simulink model "VehCtrl20260630_18B"  (R2018b)
settings: Solver=FixedStepAuto  StartTime=0.0  StopTime=inf  FixedStep=0.005  RelTol=1e-3
InitFcn:
  | mbd_mpc_consistency_checks(bdroot(gcs));
undefined symbols (not defined in the file): ANG_DEAD, BMS_NormalPwr, BrakeDeadZone, BrkPrsByBrkPct_TB_X, BrkPrsByBrkPct_TB_Y, DELAY_DISCHARGE, DELAY_RCUOFF, DRV_BACKWARD, DRV_BRAKE, DRV_FORWARD, DRV_NEUTRAL, DRV_PARK, DRV_UNPARK, DRV_ZEROTURN, EPB_LOCK, EPB_UNLOCK, ExtraLoadPwr, FanOff, fifo_0_vect, fifo_1_vect, HiFanReq, HV_finished, HV_No_Active, HV_POWER_OFF, HV_POWER_ON, HVDown, HVON, KaTLS_v_DrgUp_X_VehSpd, KeFTM_s_Way1OffDlyTime, KeFTM_TK_Way1CoolLv2OffBatTemp, KeFTM_TK_Way1CoolLv2OffMtrTemp, KeFTM_TK_Way1CoolLv2OnBatTemp, KeFTM_TK_Way1CoolLv2OnMtrTemp, KeFTM_TK_Way1CoolLv3OffBatTemp, KeFTM_TK_Way1CoolLv3OffMtrTemp, KeFTM_TK_Way1CoolLv3OnBatTemp, KeFTM_TK_Way1CoolLv3OnMtrTemp, KeFTM_TK_Way1CoolLv4OffBatTemp, KeFTM_TK_Way1CoolLv4OffMtrTemp, KeFTM_TK_Way1CoolLv4OnBatTemp, KeFTM_TK_Way1CoolLv4OnMtrTemp, Kp1, Kp2, LowFanReq, LQFP, MtrCmdGainFL, MtrCmdGainFR, MtrCmdGainRL, MtrCmdGainRR, MtrPwrFactor_RCU, MtrPwrHighToMidThd, MtrPwrLowToMidThd, MtrPwrMidToHighThd, MtrPwrMidToLowThd, MtrTrqMax, PCT_DEAD, Precharge, PTO_1000, PTO_540, pts1_fifo_0_vect ... (+32)
libraries: mbd_mpc574x_ec_toolbox x175, simulink x110, canmsglib x70
(part 7 of 15)

== system VehCtrl20260630_18B/SigOut/MCU/FL3 ==
  note: +32
  note: 0-torque
      | 1-speed
  DirCmd : Inport
  torque : Inport  Port=2
  Constant : Constant  Value=16  OutDataTypeStr=uint8
  Constant1 : Constant  Value=4  OutDataTypeStr=uint8
  Constant2 : Constant  Value=DRV_ZEROTURN  OutDataTypeStr=uint8
  Constant3 : Constant  Value=48  OutDataTypeStr=uint8
  Constant4 : Constant  Value=36  OutDataTypeStr=uint8
  Constant5 : Constant  Value=0  OutDataTypeStr=single
  Data Store Read : DataStoreRead  DataStoreName=DrvPhase
  Data Store Read1 : DataStoreRead  DataStoreName=MotorModeZeroTurn
  Data Store Read2 : DataStoreRead  DataStoreName=Gain_Trq2Spd
  GreaterThan : RelationalOperator  Operator===  OutDataTypeStr=boolean  RndMeth=Simplest
  Logical Operator : Logic  AllPortsSameDT=off  OutDataTypeStr=boolean
  NOT : Logic  Operator=NOT  IconShape=distinctive  AllPortsSameDT=off  OutDataTypeStr=boolean
  Product : Product
  Switch{,1..3} (4 alike) : Switch  Criteria=u2 > Threshold
  ModeReq : Outport
  speed : Outport  Port=2
  wires:
  DirCmd/1 -> NOT/1
  Constant/1 -> Switch/1
  Constant1/1 -> Switch/3
  Data Store Read/1 -> GreaterThan/1
  Constant2/1 -> GreaterThan/2
  GreaterThan/1 -> Logical Operator/1
  Data Store Read1/1 -> Logical Operator/2
  Logical Operator/1 -> Switch3/2, Switch1/2
  Switch/1 -> Switch1/3
  Switch1/1 -> ModeReq/1
  NOT/1 -> Switch2/2, Switch/2
  Constant4/1 -> Switch2/3
  Constant3/1 -> Switch2/1
  Switch2/1 -> Switch1/1
  torque/1 -> Product/2
  Switch3/1 -> speed/1
  Product/1 -> Switch3/1
  Data Store Read2/1 -> Product/1
  Constant5/1 -> Switch3/3

== system VehCtrl20260630_18B/SigOut/MCU/FR ==
  DirCmd : Inport
  Constant : Constant  Value=16  OutDataTypeStr=uint8
  Constant1 : Constant  Value=4  OutDataTypeStr=uint8
  NOT : Logic  Operator=NOT  IconShape=distinctive  AllPortsSameDT=off  OutDataTypeStr=boolean
  Switch : Switch  Criteria=u2 > Threshold
  ModeReq : Outport
  wires:
  Switch/1 -> ModeReq/1
  NOT/1 -> Switch/2
  Constant1/1 -> Switch/3
  Constant/1 -> Switch/1
  DirCmd/1 -> NOT/1

== system VehCtrl20260630_18B/SigOut/MCU/RL ==
  DirCmd : Inport
  Constant : Constant  Value=16  OutDataTypeStr=uint8
  Constant1 : Constant  Value=4  OutDataTypeStr=uint8
  Switch : Switch  Criteria=u2 > Threshold
  ModeReq : Outport
  wires:
  Constant/1 -> Switch/1
  Constant1/1 -> Switch/3
  DirCmd/1 -> Switch/2
  Switch/1 -> ModeReq/1

== system VehCtrl20260630_18B/SigOut/MCU/RR ==
  DirCmd : Inport
  Constant : Constant  Value=16  OutDataTypeStr=uint8
  Constant1 : Constant  Value=4  OutDataTypeStr=uint8
  NOT : Logic  Operator=NOT  IconShape=distinctive  AllPortsSameDT=off  OutDataTypeStr=boolean
  Switch : Switch  Criteria=u2 > Threshold
  ModeReq : Outport
  wires:
  Switch/1 -> ModeReq/1
  NOT/1 -> Switch/2
  Constant1/1 -> Switch/3
  Constant/1 -> Switch/1
  DirCmd/1 -> NOT/1

== system VehCtrl20260630_18B/SigOut/MCU/Subsystem ==
  <TrqCmd> : Inport
  Abs : Abs
  Add : Sum
  Constant : Constant  Value=MtrCmdGainFL
  Product : Product
  Saturation : Saturate  UpperLimit=100  LowerLimit=2
  Out1 : Outport
  wires:
  Abs/1 -> Add/1
  <TrqCmd>/1 -> Saturation/1, Abs/1
  Add/1 -> Out1/1
  Saturation/1 -> Product/1
  Product/1 -> Add/2
  Constant/1 -> Product/2  "MtrCmdGainFL"

== system VehCtrl20260630_18B/SigOut/MCU/Subsystem1 ==
  <TrqCmd> : Inport
  Abs : Abs
  Add : Sum
  Constant : Constant  Value=MtrCmdGainFR
  Product : Product
  Saturation : Saturate  UpperLimit=100  LowerLimit=2
  Out1 : Outport
  wires:
  Abs/1 -> Add/1
  <TrqCmd>/1 -> Saturation/1, Abs/1
  Add/1 -> Out1/1
  Saturation/1 -> Product/1
  Product/1 -> Add/2
  Constant/1 -> Product/2  "MtrCmdGainFR"

== system VehCtrl20260630_18B/SigOut/MCU/Subsystem2 ==
  <TrqCmd> : Inport
  Abs : Abs
  Add : Sum
  Constant : Constant  Value=MtrCmdGainRL
  Product : Product
  Saturation : Saturate  UpperLimit=100  LowerLimit=2
  Out1 : Outport
  wires:
  Abs/1 -> Add/1
  <TrqCmd>/1 -> Saturation/1, Abs/1
  Add/1 -> Out1/1
  Saturation/1 -> Product/1
  Product/1 -> Add/2
  Constant/1 -> Product/2  "MtrCmdGainRL"

== system VehCtrl20260630_18B/SigOut/MCU/Subsystem3 ==
  <TrqCmd> : Inport
  Abs : Abs
  Add : Sum
  Constant : Constant  Value=MtrCmdGainRR
  Product : Product
  Saturation : Saturate  UpperLimit=100  LowerLimit=2
  Out1 : Outport
  wires:
  Abs/1 -> Add/1
  <TrqCmd>/1 -> Saturation/1, Abs/1
  Add/1 -> Out1/1
  Saturation/1 -> Product/1
  Product/1 -> Add/2
  Constant/1 -> Product/2  "MtrCmdGainRR"

== system VehCtrl20260630_18B/SigOut/METER/Subsystem ==
  <ModeDir> : Inport
  Constant : Constant  Value=3
  Constant18 : Constant  Value=2
  Data Type Conversion : DataTypeConversion
  Data Type Conversion1 : DataTypeConversion
  Switch : Switch  Criteria=u2 > Threshold
  Out1 : Outport
  wires:
  Constant/1 -> Data Type Conversion/1
  Switch/1 -> Out1/1
  Constant18/1 -> Data Type Conversion1/1
  <ModeDir>/1 -> Switch/2
  Data Type Conversion/1 -> Switch/1
  Data Type Conversion1/1 -> Switch/3

== system VehCtrl20260630_18B/SigOut/METER/Subsystem1 ==
  <RCU_ActWorkSts> : Inport
  Constant : Constant
  Constant1 : Constant  Value=0
  Switch : Switch  Criteria=u2 > Threshold  Threshold=2
  Out1 : Outport
  wires:
  <RCU_ActWorkSts>/1 -> Switch/2
  Constant1/1 -> Switch/3
  Constant/1 -> Switch/1
  Switch/1 -> Out1/1

== system VehCtrl20260630_18B/SigOut/METER/Subsystem2 ==
  <DCDC_Optvol> : Inport
  Constant2 : Constant  Value=12.5
  Data Type Conversion : DataTypeConversion
  Equal : RelationalOperator  Operator=<=  OutDataTypeStr=boolean  RndMeth=Simplest
  Out1 : Outport
  wires:
  Constant2/1 -> Data Type Conversion/1
  Equal/1 -> Out1/1
  <DCDC_Optvol>/1 -> Equal/1
  Data Type Conversion/1 -> Equal/2

== system VehCtrl20260630_18B/SigOut/METER/Subsystem3 ==
  Constant : Constant  Value=2
  Constant1 : Constant
  Data Store Read1 : DataStoreRead  DataStoreName=CtrMode
  Data Store Read2 : DataStoreRead  DataStoreName=Fault
  Data Type Conversion : DataTypeConversion
  Data Type Conversion1 : DataTypeConversion
  Data Type Conversion2 : DataTypeConversion
  Equal : RelationalOperator  Operator===  OutDataTypeStr=boolean  RndMeth=Simplest
  Switch : Switch  Criteria=u2 > Threshold
  Out1 : Outport
  wires:
  Switch/1 -> Data Type Conversion1/1
  Data Store Read2/1 -> Switch/2
  Data Store Read1/1 -> Data Type Conversion/1
  Constant/1 -> Switch/1
  Data Type Conversion/1 -> Switch/3
  Data Type Conversion1/1 -> Equal/1
  Constant1/1 -> Data Type Conversion2/1
  Data Type Conversion2/1 -> Equal/2
  Equal/1 -> Out1/1

== system VehCtrl20260630_18B/SigOut/METER/Subsystem4 ==
  Constant : Constant  Value=2
  Constant1 : Constant  Value=0
  Data Store Read1 : DataStoreRead  DataStoreName=CtrMode
  Data Store Read2 : DataStoreRead  DataStoreName=Fault
  Data Type Conversion : DataTypeConversion
  Data Type Conversion1 : DataTypeConversion
  Data Type Conversion2 : DataTypeConversion
  Equal : RelationalOperator  Operator===  OutDataTypeStr=boolean  RndMeth=Simplest
  Switch : Switch  Criteria=u2 > Threshold
  Out1 : Outport
  wires:
  Switch/1 -> Data Type Conversion1/1
  Data Store Read2/1 -> Switch/2
  Data Store Read1/1 -> Data Type Conversion/1
  Constant/1 -> Switch/1
  Data Type Conversion/1 -> Switch/3
  Data Type Conversion1/1 -> Equal/1
  Constant1/1 -> Data Type Conversion2/1
  Data Type Conversion2/1 -> Equal/2
  Equal/1 -> Out1/1

== system VehCtrl20260630_18B/VehCtrl/EnergyManage1/Subsystem ==
  VehTrqTgt : Inport
  VehSpd : Inport  Port=2
  MCU_PTO : Inport  Port=3
  Add : Sum
  Bus Selector3 : BusSelector  OutputSignals=MCU2VCU_1.MCU_TrqEst,MCU2VCU_1.MCU_SpdEst
  Constant2 : Constant  Value=WhlRadius
  Constant3 : Constant  Value=9.55  OutDataTypeStr=single
  Divide : Product  Inputs=*/
  Divide1 : Product  Inputs=*/
  Product : Product
  Product1 : Product
  PwrCmd : Outport
  wires:
  Constant3/1 -> Divide1/2
  Divide/1 -> Product/2
  Product/1 -> Add/1
  Constant2/1 -> Divide/2
  Bus Selector3/2 -> Divide1/1  "<MCU_SpdEst>"
  Divide1/1 -> Product1/2
  Product1/1 -> Add/2
  Bus Selector3/1 -> Product1/1  "<MCU_TrqEst>"
  VehTrqTgt/1 -> Product/1
  VehSpd/1 -> Divide/1
  Add/1 -> PwrCmd/1
  MCU_PTO/1 -> Bus Selector3/1

== system VehCtrl20260630_18B/VehCtrl/FaultProc/Subsystem5 ==
  note: 1-正常
      | 0-超时
  note: 1-丢包
      | 0-正常
  AutoDrive : Inport
  Bus Selector7 : BusSelector  OutputSignals=signal1.AUTO_LiveCnt1,signal1.AUTO_CheckSum1,signal1.PacketLossFlg,signal2.AUTO_LiveCnt2,signal2.AUTO_CheckSum2,signal2.PacketLossFlg,signal3.AUTO_LiveCnt1,signal3.AUTO_CheckSum1,signal3.PacketLossFlg
  Logical Operator : Logic  Operator=NOT  AllPortsSameDT=off  OutDataTypeStr=boolean
  Logical Operator1 : Logic  Operator=OR  Inputs=3  AllPortsSameDT=off  OutDataTypeStr=boolean
  Logical Operator2 : Logic  Inputs=3  AllPortsSameDT=off  OutDataTypeStr=boolean
  PacketLoss_RMT : Stateflow chart  TreatAsAtomicUnit=on
  PacketLoss_RMT1 : Stateflow chart  TreatAsAtomicUnit=on
  PacketLoss_RMT2 : Stateflow chart  TreatAsAtomicUnit=on
  TimeOutLevel_RMT : Stateflow chart  TreatAsAtomicUnit=on
  TimeOutLevel_RMT1 : Stateflow chart  TreatAsAtomicUnit=on
  TimeOutLevel_RMT2 : Stateflow chart  TreatAsAtomicUnit=on
  TimeOut : Outport
  PacketLoss : Outport  Port=2
  wires:
  TimeOutLevel_RMT/1(TimeOutLevel) -> Logical Operator2/1  "TimeOutLevel1"
  Logical Operator2/1 -> Logical Operator/1
  [Auto_LiveCounter] -> TimeOutLevel_RMT/1(LiveCounter)
  Logical Operator1/1 -> PacketLoss/1
  [Auto_PacketLossFlg] -> PacketLoss_RMT/2(PacketLoss)
  [Auto_CheckSumFlg] -> PacketLoss_RMT/1(CheckSum)
  PacketLoss_RMT/1(PacketLossFlg) -> Logical Operator1/1
  AutoDrive/1 -> Bus Selector7/1
  Logical Operator/1 -> TimeOut/1
  [Auto_LiveCounter2] -> TimeOutLevel_RMT1/1(LiveCounter)
  TimeOutLevel_RMT1/1(TimeOutLevel) -> Logical Operator2/2  "TimeOutLevel1"
  [Auto_CheckSumFlg2] -> PacketLoss_RMT1/1(CheckSum)
  [Auto_PacketLossFlg2] -> PacketLoss_RMT1/2(PacketLoss)
  PacketLoss_RMT1/1(PacketLossFlg) -> Logical Operator1/2
  Bus Selector7/6 -> [Auto_PacketLossFlg2]  "<PacketLossFlg>"
  Bus Selector7/5 -> [Auto_CheckSumFlg2]  "<AUTO_CheckSum2>"
  Bus Selector7/4 -> [Auto_LiveCounter2]  "<AUTO_LiveCnt2>"
  Bus Selector7/3 -> [Auto_PacketLossFlg]  "<PacketLossFlg>"
  Bus Selector7/2 -> [Auto_CheckSumFlg]  "<AUTO_CheckSum1>"
  Bus Selector7/1 -> [Auto_LiveCounter]  "<AUTO_LiveCnt1>"
  Bus Selector7/7 -> [Auto_LiveCounter3]  "<AUTO_LiveCnt1>"
  Bus Selector7/8 -> [Auto_CheckSumFlg3]  "<AUTO_CheckSum1>"
  Bus Selector7/9 -> [Auto_PacketLossFlg3]  "<PacketLossFlg>"
  [Auto_LiveCounter3] -> TimeOutLevel_RMT2/1(LiveCounter)
  TimeOutLevel_RMT2/1(TimeOutLevel) -> Logical Operator2/3  "TimeOutLevel1"
  [Auto_PacketLossFlg3] -> PacketLoss_RMT2/2(PacketLoss)
  [Auto_CheckSumFlg3] -> PacketLoss_RMT2/1(CheckSum)
  PacketLoss_RMT2/1(PacketLossFlg) -> Logical Operator1/3

== system VehCtrl20260630_18B/VehCtrl/MontionControl/DriveControl ==
  EN_COM : Inport
  Ready : Inport  Port=2
  Fault : Inport  Port=3
  CMD : Inport  Port=4
  BMS : Inport  Port=5
  VehSpd : Inport  Port=6
  StrReady : Inport  Port=7
  AUTO : Inport  Port=8
  AUTOMode : Inport  Port=9
  RMT : Inport  Port=10
  DCDC : Inport  Port=11
  Brake : Subsystem
  Bus Creator{1..4} (4 alike) : BusCreator  Inputs=4
  Bus Selector : BusSelector  OutputSignals=RMT.RMT1.RMT_CmdAccPct,BrkPct,ModeDir,ModeStr,StrAng,RMT.RMT4.ModeSafety
  Constant : Constant  Value=0  OutDataTypeStr=uint8
  Constant1 : Constant
  Constant2 : Constant  Value=0  OutDataTypeStr=uint8
  Constant3 : Constant  OutDataTypeStr=boolean
  DriveModeTrans : Stateflow chart  TreatAsAtomicUnit=on
  Equal : RelationalOperator  Operator===  OutDataTypeStr=boolean  RndMeth=Simplest
  Logical Operator : Logic  AllPortsSameDT=off  OutDataTypeStr=boolean
  Motor : Subsystem
  MCUFL_OUT : Outport
  MCUFR_OUT : Outport  Port=2
  MCURL_OUT : Outport  Port=3
  MCURR_OUT : Outport  Port=4
  BrkPrsTgt : Outport  Port=5
  EpbSt : Outport  Port=6
  VehTrqTgt : Outport  Port=7
  wires:
  CMD/1 -> Bus Selector/1
  Bus Selector/3 -> DriveModeTrans/5(ModeDirection)  "<ModeDir>"
  Bus Selector/2 -> DriveModeTrans/2(CmdBrk)  "<BrkPct>"
  Brake/1(BrkPrsTgt) -> BrkPrsTgt/1
  DriveModeTrans/1(VehBrk) -> Brake/1(VehBrkTgt)
  DriveModeTrans/2(EpbSt) -> EpbSt/1
  VehSpd/1 -> DriveModeTrans/9(VehSpd), Motor/5(VehSpd)
  DriveModeTrans/3(VehDrv) -> Motor/1(VehDrvPct)
  Bus Selector/1 -> DriveModeTrans/1(CmdDrv)  "<RMT_CmdAccPct>"
  Bus Selector/4 -> Logical Operator/1  "<ModeStr>"
  StrReady/1 -> DriveModeTrans/8(StrReady)
  DriveModeTrans/4(SpdTgt) -> Motor/2(CmdSpd)
  DriveModeTrans/5(ModeSpd) -> Motor/3(ModeSpeed)
  DriveModeTrans/6(DrvPhase) -> Motor/4(DrvPhase)
  Bus Selector/5 -> Motor/6(CmdStrAng)  "<StrAng>"
  Motor/2(MtrDirCmdFL) -> Bus Creator1/2  "DirCmd"
  Motor/1(Enable) -> Bus Creator1/1, Bus Creator2/1, Bus Creator4/1, Bus Creator3/1  "Enable"
  Bus Creator4/1 -> MCURR_OUT/1
  Bus Creator2/1 -> MCUFR_OUT/1
  Motor/13(MtrSpdCmdRR) -> Bus Creator4/4  "SpdCmd"
  Motor/12(MtrTrqCmdRR) -> Bus Creator4/3  "TrqCmd"
  Motor/11(MtrDirCmdRR) -> Bus Creator4/2  "DirCmd"
  Bus Creator1/1 -> MCUFL_OUT/1
  Motor/7(MtrSpdCmdFR) -> Bus Creator2/4  "SpdCmd"
  Motor/6(MtrTrqCmdFR) -> Bus Creator2/3  "TrqCmd"
  Bus Creator3/1 -> MCURL_OUT/1
  Motor/10(MtrSpdCmdRL) -> Bus Creator3/4  "SpdCmd"
  Motor/4(MtrSpdCmdFL) -> Bus Creator1/4  "SpdCmd"
  Motor/9(MtrTrqCmdRL) -> Bus Creator3/3  "TrqCmd"
  Motor/3(MtrTrqCmdFL) -> Bus Creator1/3  "TrqCmd"
  Motor/8(MtrDirCmdRL) -> Bus Creator3/2  "DirCmd"
  Motor/5(MtrDirCmdFR) -> Bus Creator2/2  "DirCmd"
  Ready/1 -> Motor/9(Ready)
  Motor/14(VehTrqTgt) -> VehTrqTgt/1
  Constant/1 -> DriveModeTrans/3(ModeDrive)
  Constant1/1 -> DriveModeTrans/4(CmdPark)
  Constant2/1 -> DriveModeTrans/7(CmdSpd)
  Bus Selector/6 -> Equal/1, Motor/7(ModeSafety)  "<ModeSafety>"
  AUTO/1 -> Motor/10(AUTO)
  AUTOMode/1 -> Motor/11(AUTOMode)
  BMS/1 -> Motor/12(BMS)
  RMT/1 -> Motor/13(RMT)
  DCDC/1 -> Motor/14(DCDC)
  Fault/1 -> Brake/2(In2), Motor/8(Fault)
  Logical Operator/1 -> DriveModeTrans/6(ModeSteer)
  Equal/1 -> Logical Operator/2
  Constant3/1 -> Equal/2
  EN_COM/1 -> Motor/15(EN_COM)

== system VehCtrl20260630_18B/VehCtrl/MontionControl/PtoControl ==
  CMD : Inport
  Fault : Inport  Port=2
  Ready : Inport  Port=3
  AUTOMode : Inport  Port=4
  AUTO : Inport  Port=5
  Bus Creator : BusCreator  Inputs=4
  Bus Selector : BusSelector  OutputSignals=ShutDown,NonDrive,NonPto
  Bus Selector1 : BusSelector  OutputSignals=RMT.RMT4.RMT_PtoMode
  Bus Selector2 : BusSelector  OutputSignals=signal2.AUTO_PtoSpd
  Constant5 : Constant  Value=0  OutDataTypeStr=single
  Constant6 : Constant  OutDataTypeStr=uint8
  Constant7 : Constant  Value=0  OutDataTypeStr=uint8
  Logical Operator : Logic  Operator=OR  Inputs=3  AllPortsSameDT=off  OutDataTypeStr=boolean
  Logical Operator1 : Logic  AllPortsSameDT=off  OutDataTypeStr=boolean
  NOT : Logic  Operator=NOT  IconShape=distinctive  AllPortsSameDT=off  OutDataTypeStr=boolean
  Subsystem : Subsystem
  Subsystem1 : Subsystem
  Switch2 : Switch  Criteria=u2 > Threshold
  MCU_PTO_OUT : Outport
  wires:
  CMD/1 -> Bus Selector1/1
  Constant5/1 -> Bus Creator/3  "MtrTrqCmd"
  Subsystem/1(ModeReq) -> Bus Creator/1  "ModeReq"
  Constant6/1 -> Subsystem/1(ModeSpeed)
  Constant7/1 -> Subsystem/2(DirCmd)
  Fault/1 -> Bus Selector/1
  Bus Selector/1 -> Logical Operator/1  "<ShutDown>"
  Bus Selector/2 -> Logical Operator/2  "<NonDrive>"
  Bus Selector/3 -> Logical Operator/3  "<NonPto>"
  Logical Operator/1 -> NOT/1
  Ready/1 -> Logical Operator1/2
  NOT/1 -> Logical Operator1/1
  Logical Operator1/1 -> Bus Creator/4  "Enable"
  Bus Creator/1 -> MCU_PTO_OUT/1
  AUTOMode/1 -> Switch2/2
  Bus Selector1/1 -> Subsystem1/1(<RMT_PtoMode>)  "<RMT_PtoMode>"
  AUTO/1 -> Bus Selector2/1
  Bus Selector2/1 -> Switch2/1  "<AUTO_PtoSpd>"
  Switch2/1 -> Bus Creator/2  "MtrSpdCmd"
  Subsystem1/1(MtrSpdCmd) -> Switch2/3

== system VehCtrl20260630_18B/VehCtrl/MontionControl/SteerControl ==
  note: 这个是模式，不是方向
  VehSpd : Inport
  CMD : Inport  Port=2
  BDX : Inport  Port=3
  Bus Selector : BusSelector  OutputSignals=ModeStr,StrAng
  Bus Selector1 : BusSelector  OutputSignals=AVCU.BDX_SteeringAngle
  Chart : Stateflow chart  TreatAsAtomicUnit=on
  Constant2 : Constant  Value=10  OutDataTypeStr=uint8
  GreaterThan : RelationalOperator  Operator=<  OutDataTypeStr=boolean  RndMeth=Simplest
  StrReady : Outport
  AngCmd : Outport  Port=2
  wires:
  CMD/1 -> Bus Selector/1
  Bus Selector/1 -> Chart/2(Mode)  "<ModeStr>"
  Bus Selector/2 -> Chart/3(AngCmd)  "<StrAng>"
  BDX/1 -> Bus Selector1/1
  Bus Selector1/1 -> Chart/4(Ang)  "<BDX_SteeringAngle>"
  Chart/2(StrPhase) -> GreaterThan/1
  GreaterThan/1 -> StrReady/1
  Constant2/1 -> GreaterThan/2
  VehSpd/1 -> Chart/1(VehSpd)
  Chart/1(AngCmdOut) -> AngCmd/1

== system VehCtrl20260630_18B/VehCtrl/MontionControl/ValveControl ==
  note: 仅在安全模式下才能控制
  BrkPrsTgt : Inport
  EpbSt : Inport  Port=2
  BDX : Inport  Port=3
  CMD : Inport  Port=4
  Ready : Inport  Port=5
  "AngCmd " : Inport  Port=6
  fault : Inport  Port=7
  VehSpd : Inport  Port=8
  BrakeSys : Subsystem
  Bus Creator : BusCreator  Inputs=9
  Bus Selector : BusSelector  OutputSignals=ModeSusp,RMT.RMT4.ModeSafety,RMT.RMT2.RMT_ModeWidth
  Bus Selector1 : BusSelector  OutputSignals=AVCU.BDX_BrakePressure
  Bus Selector2 : BusSelector  OutputSignals=NonDrive
  EpbSys : Subsystem
  PumpSys : Subsystem
  SteerSys : Subsystem
  SuspesionSys : Subsystem
  WidthSys : Subsystem
  BDX_OUT : Outport
  wires:
  CMD/1 -> Bus Selector/1
  BDX/1 -> Bus Selector1/1
  BrkPrsTgt/1 -> BrakeSys/1(BrkPrsTgt)
  Bus Selector1/1 -> BrakeSys/2(BrkPrs)  "<BDX_BrakePressure>"
  Bus Selector/1 -> SuspesionSys/1(SuspSt)  "<ModeSusp>"
  Bus Selector/3 -> WidthSys/2(<RMT_ModeWidth>)  "<RMT_ModeWidth>"
  BrakeSys/1(BrkValve) -> Bus Creator/2  "BrkValve"
  SuspesionSys/1(SuspUpValve) -> Bus Creator/6  "SuspUpValve"
  PumpSys/1(Pump) -> Bus Creator/1  "Pump"
  EpbSys/1(EpbValve) -> Bus Creator/5  "EpbValve"
  SteerSys/1(SteerValveL) -> Bus Creator/3  "SteerValveL"
  WidthSys/1(WidthLengthenValve) -> Bus Creator/8  "WidthLengthenValve"
  WidthSys/2(WidthShortenValve) -> Bus Creator/9  "WidthShortenValve"
  Bus Creator/1 -> BDX_OUT/1
  SteerSys/2(SteerValveR) -> Bus Creator/4  "SteerValveR"
  EpbSt/1 -> EpbSys/1(EpbSt)
  SuspesionSys/2(SuspDownValve) -> Bus Creator/7  "SuspDownValve"
  Ready/1 -> PumpSys/1(Ready)
  Bus Selector/2 -> WidthSys/1(ModeSafety), SuspesionSys/2(ModeSafety)  "<ModeSafety>"
  fault/1 -> Bus Selector2/1
  Bus Selector2/1 -> SteerSys/2(In2)  "<NonDrive>"
  VehSpd/1 -> SteerSys/3(VehSpd)
  "AngCmd "/1 -> SteerSys/1(AngCmd)

== system VehCtrl20260630_18B/VehCtrl/TempertureControl/Lv_to_Dut1 ==
  note: 就是整型，不要替换为single
  MCUReqMtrPumpLv : Inport
  2-D Lookup Table1 : Lookup_n-D  NumberOfTableDimensions=1  BreakpointsForDimension1=uint8([ 0 1 2 3 4 ])  BreakpointsForDimension2=KaTLS_v_DrgUp_X_VehSpd  Table=uint16([ 5 30 40 55 70])  TableDataTypeStr=uint16  ExtrapMethod=Clip  UseLastTableValue=on  OutDataTypeStr=Inherit: Inherit from 'Table data'  RndMeth=Simplest
  Gain : Gain  Gain=1/100  OutDataTypeStr=single
  MCUReqMtrPumpDut : Outport
  wires:
  MCUReqMtrPumpLv/1 -> 2-D Lookup Table1/1
  2-D Lookup Table1/1 -> Gain/1
  Gain/1 -> MCUReqMtrPumpDut/1

== system VehCtrl20260630_18B/VehCtrl/TempertureControl/Lv_to_Dut2 ==
  note: 就是整型，不要替换为single
  MCUReqMtrPumpLv : Inport
  2-D Lookup Table1 : Lookup_n-D  NumberOfTableDimensions=1  BreakpointsForDimension1=uint8([ 0 1 2 3 4 ])  BreakpointsForDimension2=KaTLS_v_DrgUp_X_VehSpd  Table=uint16([ 5 30 40 55 70])  TableDataTypeStr=uint16  ExtrapMethod=Clip  UseLastTableValue=on  OutDataTypeStr=Inherit: Inherit from 'Table data'  RndMeth=Simplest
  Gain : Gain  Gain=1/100  OutDataTypeStr=single
  MCUReqMtrPumpDut : Outport
  wires:
  MCUReqMtrPumpLv/1 -> 2-D Lookup Table1/1
  2-D Lookup Table1/1 -> Gain/1
  Gain/1 -> MCUReqMtrPumpDut/1

== system VehCtrl20260630_18B/VehCtrl/TempertureControl/Lv_to_Dut3 ==
  note: 就是整型，不要替换为single
  MCUReqBatPumpLv : Inport
  2-D Lookup Table1 : Lookup_n-D  NumberOfTableDimensions=1  BreakpointsForDimension1=uint8([ 0 1 2 3 4 ])  BreakpointsForDimension2=KaTLS_v_DrgUp_X_VehSpd  Table=uint16([ 5 30 40 55 70])  TableDataTypeStr=uint16  ExtrapMethod=Clip  UseLastTableValue=on  OutDataTypeStr=Inherit: Inherit from 'Table data'  RndMeth=Simplest
  Gain : Gain  Gain=1/100  OutDataTypeStr=single
  MCUReqBatPumpDut : Outport
  wires:
  MCUReqBatPumpLv/1 -> 2-D Lookup Table1/1
  2-D Lookup Table1/1 -> Gain/1
  Gain/1 -> MCUReqBatPumpDut/1

== system VehCtrl20260630_18B/VehCtrl/TempertureControl/ThermFR_RRvRead1 ==
  RdySt : Inport
  MtrTemp : Inport  Port=2
  Cnt_To_s : Subsystem
  Constant10 : Constant  Value=KeFTM_TK_Way1CoolLv3OnMtrTemp
  Constant11 : Constant  Value=KeFTM_TK_Way1CoolLv2OffMtrTemp
  Constant12 : Constant  Value=KeFTM_TK_Way1CoolLv2OnMtrTemp
  Constant13 : Constant  Value=KeFTM_TK_Way1CoolLv4OnMtrTemp
  Constant7 : Constant  Value=KeFTM_s_Way1OffDlyTime
  Constant8 : Constant  Value=KeFTM_TK_Way1CoolLv4OffMtrTemp
  Constant9 : Constant  Value=KeFTM_TK_Way1CoolLv3OffMtrTemp
  Way1_Cool_Level : Stateflow chart  TreatAsAtomicUnit=on
  MtrPumpLvReq : Outport
  Fan_Low : Outport  Port=2
  wires:
  Way1_Cool_Level/2(MtrPumpLv) -> MtrPumpLvReq/1  "MtrPumpLvReq2"
  Way1_Cool_Level/1(Fan_Low) -> Fan_Low/1  "FanLvReq2"
  RdySt/1 -> Way1_Cool_Level/1(RdySt)
  Constant13/1 -> Way1_Cool_Level/8(Ke_Lv4OnTemp)
  Constant12/1 -> Way1_Cool_Level/4(Ke_Lv2OnTemp)
  Constant10/1 -> Way1_Cool_Level/6(Ke_Lv3OnTemp)
  Constant9/1 -> Way1_Cool_Level/5(Ke_Lv3OffTemp)
  Constant11/1 -> Way1_Cool_Level/3(Ke_Lv2OffTemp)
  Constant7/1 -> Cnt_To_s/1(In1)
  Constant8/1 -> Way1_Cool_Level/7(Ke_Lv4OffTemp)
  Cnt_To_s/1(Out1) -> Way1_Cool_Level/9(Ke_OffDlyCnt)
  MtrTemp/1 -> Way1_Cool_Level/2(Temp)

== system VehCtrl20260630_18B/VehCtrl/TempertureControl/ThermFR_RRvRead2 ==
  RdySt : Inport
  MtrTemp : Inport  Port=2
  Cnt_To_s : Subsystem
  Constant10 : Constant  Value=KeFTM_TK_Way1CoolLv3OnMtrTemp
  Constant11 : Constant  Value=KeFTM_TK_Way1CoolLv2OffMtrTemp
  Constant12 : Constant  Value=KeFTM_TK_Way1CoolLv2OnMtrTemp
  Constant13 : Constant  Value=KeFTM_TK_Way1CoolLv4OnMtrTemp
  Constant7 : Constant  Value=KeFTM_s_Way1OffDlyTime
  Constant8 : Constant  Value=KeFTM_TK_Way1CoolLv4OffMtrTemp
  Constant9 : Constant  Value=KeFTM_TK_Way1CoolLv3OffMtrTemp
  Way1_Cool_Level : Stateflow chart  TreatAsAtomicUnit=on
  MtrPumpLvReq : Outport
  Fan_Low : Outport  Port=2
  wires:
  MtrTemp/1 -> Way1_Cool_Level/2(Temp)
  Cnt_To_s/1(Out1) -> Way1_Cool_Level/9(Ke_OffDlyCnt)
  Constant8/1 -> Way1_Cool_Level/7(Ke_Lv4OffTemp)
  Constant7/1 -> Cnt_To_s/1(In1)
  Constant11/1 -> Way1_Cool_Level/3(Ke_Lv2OffTemp)
  Constant9/1 -> Way1_Cool_Level/5(Ke_Lv3OffTemp)
  Constant10/1 -> Way1_Cool_Level/6(Ke_Lv3OnTemp)
  Constant12/1 -> Way1_Cool_Level/4(Ke_Lv2OnTemp)
  Constant13/1 -> Way1_Cool_Level/8(Ke_Lv4OnTemp)
  RdySt/1 -> Way1_Cool_Level/1(RdySt)
  Way1_Cool_Level/1(Fan_Low) -> Fan_Low/1  "FanLvReq2"
  Way1_Cool_Level/2(MtrPumpLv) -> MtrPumpLvReq/1  "MtrPumpLvReq2"

== system VehCtrl20260630_18B/VehCtrl/TempertureControl/ThermLvRead3 ==
  RdySt : Inport
  Temp : Inport  Port=2
  Cnt_To_s : Subsystem
  Constant10 : Constant  Value=KeFTM_TK_Way1CoolLv3OnBatTemp
  Constant11 : Constant  Value=KeFTM_TK_Way1CoolLv2OffBatTemp
  Constant12 : Constant  Value=KeFTM_TK_Way1CoolLv2OnBatTemp
  Constant13 : Constant  Value=KeFTM_TK_Way1CoolLv4OnBatTemp
  Constant7 : Constant  Value=KeFTM_s_Way1OffDlyTime
  Constant8 : Constant  Value=KeFTM_TK_Way1CoolLv4OffBatTemp
  Constant9 : Constant  Value=KeFTM_TK_Way1CoolLv3OffBatTemp
  Way1_Cool_Level : Stateflow chart  TreatAsAtomicUnit=on
  Fan_Low : Outport
  Fan_High : Outport  Port=2
  v1 : Outport  Port=3
  v2 : Outport  Port=4
  v3 : Outport  Port=5
  v4 : Outport  Port=6
  PumpLvReq : Outport  Port=7
  wires:
  Way1_Cool_Level/2(Fan_High) -> Fan_High/1
  Temp/1 -> Way1_Cool_Level/2(Temp)
  RdySt/1 -> Way1_Cool_Level/1(RdySt)
  Constant13/1 -> Way1_Cool_Level/8(Ke_Lv4OnTemp)
  Constant9/1 -> Way1_Cool_Level/5(Ke_Lv3OffTemp)
  Constant12/1 -> Way1_Cool_Level/4(Ke_Lv2OnTemp)
  Constant10/1 -> Way1_Cool_Level/6(Ke_Lv3OnTemp)
  Constant7/1 -> Cnt_To_s/1(In1)
  Constant8/1 -> Way1_Cool_Level/7(Ke_Lv4OffTemp)
  Cnt_To_s/1(Out1) -> Way1_Cool_Level/9(Ke_OffDlyCnt)
  Constant11/1 -> Way1_Cool_Level/3(Ke_Lv2OffTemp)
  Way1_Cool_Level/7(MtrPumpLv) -> PumpLvReq/1  "MtrPumpLvReq2"
  Way1_Cool_Level/1(Fan_Low) -> Fan_Low/1  "FanLvReq2"
  Way1_Cool_Level/3(V1) -> v1/1
  Way1_Cool_Level/4(V2) -> v2/1
  Way1_Cool_Level/5(V3) -> v3/1
  Way1_Cool_Level/6(V4) -> v4/1

== system VehCtrl20260630_18B/Initialization & SPI timer1/CS1 LS/Subsystem/SPI_en ==
  Action Port : ActionPort
  Add : Sum
  Add1 : Sum  Inputs=+++
  Constant1 : Constant  Value=0
  Constant11 : Constant  OutDataTypeStr=uint8
  Constant2 : Constant  OutDataTypeStr=uint8
  Constant3 : Constant  Value=0
  Constant9 : Constant  Value=128  OutDataTypeStr=uint8
  Data Type Conversion : DataTypeConversion
  Data Type Conversion1 : DataTypeConversion
  Gain : Gain  Gain=64
  Out1 : Outport
  Out2 : Outport  Port=2
  wires:
  Constant1/1 -> Add/1
  Constant9/1 -> Add1/1
  Add1/1 -> Data Type Conversion/1
  Constant11/1 -> Add1/2
  Constant2/1 -> Gain/1
  Gain/1 -> Add1/3
  Add/1 -> Data Type Conversion1/1
  Constant3/1 -> Add/2
  Data Type Conversion/1 -> Out1/1
  Data Type Conversion1/1 -> Out2/1

== system VehCtrl20260630_18B/Initialization & SPI timer1/CS1 LS/Subsystem/clear  ==
  Action Port : ActionPort
  Add : Sum
  Add1 : Sum  Inputs=+++
  Constant1 : Constant
  Constant11 : Constant  Value=7  OutDataTypeStr=uint8
  Constant2 : Constant  Value=0  OutDataTypeStr=uint8
  Constant3 : Constant  Value=0
  Constant9 : Constant  Value=128  OutDataTypeStr=uint8
  Data Type Conversion : DataTypeConversion
  Data Type Conversion1 : DataTypeConversion
  Gain : Gain  Gain=64
  Out1 : Outport
  Out2 : Outport  Port=2
  wires:
  Constant3/1 -> Add/2
  Add/1 -> Data Type Conversion1/1
  Gain/1 -> Add1/3
  Constant2/1 -> Gain/1
  Constant11/1 -> Add1/2
  Add1/1 -> Data Type Conversion/1
  Data Type Conversion1/1 -> Out2/1
  Data Type Conversion/1 -> Out1/1
  Constant9/1 -> Add1/1
  Constant1/1 -> Add/1

== system VehCtrl20260630_18B/Initialization & SPI timer1/CS1 LS/Subsystem/confi_enbit ==
  Action Port : ActionPort
  Add : Sum
  Add1 : Sum  Inputs=+++
  Constant1 : Constant
  Constant11 : Constant  Value=7  OutDataTypeStr=uint8
  Constant2 : Constant  OutDataTypeStr=uint8
  Constant3 : Constant  Value=128
  Constant9 : Constant  Value=128  OutDataTypeStr=uint8
  Data Type Conversion : DataTypeConversion
  Data Type Conversion1 : DataTypeConversion
  Gain : Gain  Gain=64
  Out1 : Outport
  Out2 : Outport  Port=2
  wires:
  Constant1/1 -> Add/1
  Constant9/1 -> Add1/1
  Add1/1 -> Data Type Conversion/1
  Constant11/1 -> Add1/2
  Constant2/1 -> Gain/1
  Gain/1 -> Add1/3
  Add/1 -> Data Type Conversion1/1
  Constant3/1 -> Add/2
  Data Type Conversion/1 -> Out1/1
  Data Type Conversion1/1 -> Out2/1

== system VehCtrl20260630_18B/Initialization & SPI timer1/CS3 LS/Subsystem/A组配置 ==
  Action Port : ActionPort
  Add : Sum  Inputs=+++
  Add1 : Sum  Inputs=+++
  Bias : Bias  Bias=1
  Constant : Constant
  Constant10 : Constant  Value=2
  Constant9 : Constant  Value=80  OutDataTypeStr=uint8
  Data Store Read1 : DataStoreRead  DataStoreName=cnt2
  Data Store Write : DataStoreWrite  DataStoreName=SPI3_CTRL1
  Data Store Write1 : DataStoreWrite  DataStoreName=cnt2
  Data Type Conversion : DataTypeConversion  OutDataTypeStr=uint8
  Data Type Conversion1 : DataTypeConversion  OutDataTypeStr=uint8
  Data Type Conversion2 : DataTypeConversion
  Gain : Gain  Gain=4
  Gain1 : Gain
  Gain2 : Gain  Gain=4
  Gain3 : Gain
  Manual Switch : ManualSwitch  CurrentSetting=0
  PIN : Constant  Value=2
  SPI : Constant  Value=0
  Switch4 : Switch  Criteria=u2 > Threshold  Threshold=2
  default SPI : Constant  Value=0
  Out1 : Outport  VectorParamsAs1DForOutWhenUnconnected=on
  Out2 : Outport  Port=2  VectorParamsAs1DForOutWhenUnconnected=on
  wires:
  Switch4/1 -> Data Type Conversion2/1
  Constant/1 -> Switch4/3
  Constant10/1 -> Switch4/1
  Data Store Read1/1 -> Bias/1
  Bias/1 -> Data Store Write1/1, Switch4/2
  Data Type Conversion2/1 -> Data Store Write/1
  Data Type Conversion/1 -> Out1/1
  Data Type Conversion1/1 -> Out2/1
  Constant9/1 -> Add1/1
  Add/1 -> Data Type Conversion1/1
  [Mode] -> Gain3/1, Gain2/1, Gain1/1, Gain/1
  Gain2/1 -> Add/1
  Gain3/1 -> Add/2
  default SPI/1 -> Add/3
  Add1/1 -> Data Type Conversion/1
  Gain/1 -> Add1/2
  Gain1/1 -> Add1/3
  SPI/1 -> Manual Switch/1
  Manual Switch/1 -> [Mode]
  PIN/1 -> Manual Switch/2

== system VehCtrl20260630_18B/Initialization & SPI timer1/CS3 LS/Subsystem/B组配置 ==
  Action Port : ActionPort
  Bias : Bias  Bias=1
  Constant : Constant  Value=2
  Constant1 : Constant  Value=0  OutDataTypeStr=uint8
  Constant10 : Constant  Value=3
  Constant9 : Constant  Value=96  OutDataTypeStr=uint8
  Data Store Read1 : DataStoreRead  DataStoreName=cnt2
  Data Store Write : DataStoreWrite  DataStoreName=SPI3_CTRL1
  Data Store Write1 : DataStoreWrite  DataStoreName=cnt2
  Data Type Conversion : DataTypeConversion  OutDataTypeStr=uint8
  Data Type Conversion1 : DataTypeConversion  OutDataTypeStr=uint8
  Data Type Conversion2 : DataTypeConversion
  Switch4 : Switch  Criteria=u2 > Threshold  Threshold=4
  Out1 : Outport  VectorParamsAs1DForOutWhenUnconnected=on
  Out2 : Outport  Port=2  VectorParamsAs1DForOutWhenUnconnected=on
  wires:
  Data Type Conversion2/1 -> Data Store Write/1
  Bias/1 -> Switch4/2, Data Store Write1/1
  Data Store Read1/1 -> Bias/1
  Constant10/1 -> Switch4/1
  Constant/1 -> Switch4/3
  Switch4/1 -> Data Type Conversion2/1
  Constant1/1 -> Data Type Conversion1/1
  Data Type Conversion/1 -> Out1/1
  Constant9/1 -> Data Type Conversion/1
  Data Type Conversion1/1 -> Out2/1

== system VehCtrl20260630_18B/Initialization & SPI timer1/CS5 LS/Subsystem/SPI_en ==
  Action Port : ActionPort
  Add : Sum
  Add1 : Sum  Inputs=+++
  Constant1 : Constant  Value=0
  Constant11 : Constant  OutDataTypeStr=uint8
  Constant2 : Constant  OutDataTypeStr=uint8
  Constant3 : Constant  Value=0
  Constant9 : Constant  Value=128  OutDataTypeStr=uint8
  Data Type Conversion : DataTypeConversion
  Data Type Conversion1 : DataTypeConversion
  Gain : Gain  Gain=64
  Out1 : Outport
  Out2 : Outport  Port=2
  wires:
  Constant1/1 -> Add/1
  Constant9/1 -> Add1/1
  Add1/1 -> Data Type Conversion/1
  Constant11/1 -> Add1/2
  Constant2/1 -> Gain/1
  Gain/1 -> Add1/3
  Add/1 -> Data Type Conversion1/1
  Constant3/1 -> Add/2
  Data Type Conversion/1 -> Out1/1
  Data Type Conversion1/1 -> Out2/1

== system VehCtrl20260630_18B/Initialization & SPI timer1/CS5 LS/Subsystem/clear  ==
  Action Port : ActionPort
  Add : Sum
  Add1 : Sum  Inputs=+++
  Constant1 : Constant
  Constant11 : Constant  Value=7  OutDataTypeStr=uint8
  Constant2 : Constant  Value=0  OutDataTypeStr=uint8
  Constant3 : Constant  Value=0
  Constant9 : Constant  Value=128  OutDataTypeStr=uint8
  Data Type Conversion : DataTypeConversion
  Data Type Conversion1 : DataTypeConversion
  Gain : Gain  Gain=64
  Out1 : Outport
  Out2 : Outport  Port=2
  wires:
  Constant3/1 -> Add/2
  Add/1 -> Data Type Conversion1/1
  Gain/1 -> Add1/3
  Constant2/1 -> Gain/1
  Constant11/1 -> Add1/2
  Add1/1 -> Data Type Conversion/1
  Data Type Conversion1/1 -> Out2/1
  Data Type Conversion/1 -> Out1/1
  Constant9/1 -> Add1/1
  Constant1/1 -> Add/1

== system VehCtrl20260630_18B/Initialization & SPI timer1/CS5 LS/Subsystem/confi_enbit ==
  Action Port : ActionPort
  Add : Sum
  Add1 : Sum  Inputs=+++
  Constant1 : Constant
  Constant11 : Constant  Value=7  OutDataTypeStr=uint8
  Constant2 : Constant  OutDataTypeStr=uint8
  Constant3 : Constant  Value=128
  Constant9 : Constant  Value=128  OutDataTypeStr=uint8
  Data Type Conversion : DataTypeConversion
  Data Type Conversion1 : DataTypeConversion
  Gain : Gain  Gain=64
  Out1 : Outport
  Out2 : Outport  Port=2
  wires:
  Constant1/1 -> Add/1
  Constant9/1 -> Add1/1
  Add1/1 -> Data Type Conversion/1
  Constant11/1 -> Add1/2
  Constant2/1 -> Gain/1
  Gain/1 -> Add1/3
  Add/1 -> Data Type Conversion1/1
  Constant3/1 -> Add/2
  Data Type Conversion/1 -> Out1/1
  Data Type Conversion1/1 -> Out2/1

== system VehCtrl20260630_18B/SigIn/CAN0/AUTO1/UNPACK ==
  ID : Inport
  data : Inport  Port=2
  length : Inport  Port=3
  timestamp : Inport  Port=4
  Action Port : ActionPort  ActionType=case
  Add : Sum
  Add1 : Sum  Inputs=+-
  Auto PacketLoss : Stateflow chart  TreatAsAtomicUnit=on
  Bitwise XOR : simulink/Logic and Bit Operations/Bitwise Operator  logicop=XOR  UseBitMask=off  NumInputPorts=7  BitMask=bin2dec('11011001')  BitMaskRealWorld=Stored Integer
  Bus Creator : BusCreator  Inputs=7  OutDataTypeStr=Bus: CAN_MESSAGE_BUS  NonVirtualBus=on
  Bus Creator2 : BusCreator  Inputs=8
  Bus Selector : BusSelector  OutputSignals=AUTO_LiveCnt1
  Bus Selector1 : BusSelector  OutputSignals=AUTO_BrkPdlPct,AUTO_CheckSum1,AUTO_CtrlMode,AUTO_LiveCnt1,AUTO_ShiftSt,AUTO_StrAng,AUTO_StrMode
  Compare To Constant : simulink/Logic and Bit Operations/Compare To Constant  relop=>=  const=1  OutDataTypeStr=boolean
  Constant : Constant  OutDataTypeStr=uint8
  Constant1 : Constant  OutDataTypeStr=uint8
  Constant2 : Constant  Value=0
  Constant4 : Constant  Value=0  OutDataTypeStr=uint8
  Constant5 : Constant  Value=0  OutDataTypeStr=uint8
  Data Store Read : DataStoreRead  DataStoreName=Cnt_AUTO1
  Data Store Write : DataStoreWrite  DataStoreName=Cnt_AUTO1
  Data Type Conversion{,14..15,17} (4 alike) : DataTypeConversion  OutDataTypeStr=uint8
  Data Type Conversion1 : DataTypeConversion
  Data Type Conversion18 : DataTypeConversion  OutDataTypeStr=uint32
  Data Type Conversion19 : DataTypeConversion  OutDataTypeStr=double
  Demux : Demux  Outputs=8
  If : If
  If Action Subsystem : Subsystem  TreatAsAtomicUnit=on
  Manual Switch : ManualSwitch
  Merge : Merge
  Subsystem : Subsystem
  Unit Delay : UnitDelay  SampleTime=-1
  Message : Outport
  wires:
  Constant4/1 -> Data Type Conversion15/1
  length/1 -> Data Type Conversion14/1
  Data Type Conversion18/1 -> Bus Creator/5  "ID"
  Constant1/1 -> Data Type Conversion/1
  Constant5/1 -> Data Type Conversion17/1
  ID/1 -> Data Type Conversion18/1
  Data Type Conversion19/1 -> Bus Creator/6  "Timestamp"
  timestamp/1 -> Data Type Conversion19/1
  Data Type Conversion17/1 -> Bus Creator/4  "Error"
  Data Type Conversion/1 -> Bus Creator/1  "Extended"
  Data Type Conversion14/1 -> Bus Creator/2  "Length"
  Data Type Conversion15/1 -> Bus Creator/3  "Remote"
  Data Store Read/1 -> Add/1
  Constant/1 -> Add/2
  Add/1 -> Data Store Write/1
  Demux/2 -> Bitwise XOR/2
  Bitwise XOR/1 -> Add1/1
  Demux/4 -> Bitwise XOR/4
  Demux/8 -> Add1/2
  Add1/1 -> Compare To Constant/1
  Demux/3 -> Bitwise XOR/3
  Demux/7 -> Bitwise XOR/7
  Demux/6 -> Bitwise XOR/6
  Manual Switch/1 -> [checkSumFlg]
  data/1 -> Demux/1, Bus Creator/7  "Data"
  Demux/5 -> Bitwise XOR/5
  Demux/1 -> Bitwise XOR/1
  If/1 -> If Action Subsystem/Action
  Unit Delay/1 -> If Action Subsystem/1(In1)
  Subsystem/1(Out1) -> Merge/2
  Bus Selector/1 -> [LiveCounter]  "<AUTO_LiveCnt1>"
  If Action Subsystem/1(Out1) -> Merge/1
  If/2 -> Subsystem/Action
  [checkSumFlg] -> Data Type Conversion1/1
  Data Type Conversion1/1 -> If/1
  Merge/1 -> Bus Selector1/1, Unit Delay/1, Bus Selector/1
  Bus Selector1/1 -> Bus Creator2/1  "<AUTO_BrkPdlPct>"
  Bus Selector1/2 -> Bus Creator2/2  "<AUTO_CheckSum1>"
  Bus Selector1/3 -> Bus Creator2/3  "<AUTO_CtrlMode>"
  Bus Selector1/4 -> Bus Creator2/4  "<AUTO_LiveCnt1>"
  Bus Selector1/5 -> Bus Creator2/5  "<AUTO_ShiftSt>"
  Bus Selector1/6 -> Bus Creator2/6  "<AUTO_StrAng>"
  Bus Selector1/7 -> Bus Creator2/7  "<AUTO_StrMode>"
  Auto PacketLoss/1(PacketLossFlg) -> [PacketLossFlg]  "PacketLossFlg"
  [checkSumFlg] -> Auto PacketLoss/2(CheckSumFlg)
  [LiveCounter] -> Auto PacketLoss/1(LiveCnt)
  Bus Creator2/1 -> Message/1
  [PacketLossFlg] -> Bus Creator2/8  "PacketLossFlg"
  [checkSumFlg] -> Subsystem/1(In1)
  Bus Creator/1 -> Subsystem/2(CAN_Msg_In)  "CAN_Msg_In"
  Constant2/1 -> Manual Switch/1
  Compare To Constant/1 -> Manual Switch/2

== system VehCtrl20260630_18B/SigIn/CAN0/AUTO2/UNPACK ==
  ID : Inport
  data : Inport  Port=2
  length : Inport  Port=3
  timestamp : Inport  Port=4
  Action Port : ActionPort  ActionType=case
  Add : Sum
  Add1 : Sum  Inputs=+-
  Auto PacketLoss : Stateflow chart  TreatAsAtomicUnit=on
  Bitwise XOR : simulink/Logic and Bit Operations/Bitwise Operator  logicop=XOR  UseBitMask=off  NumInputPorts=7  BitMask=bin2dec('11011001')  BitMaskRealWorld=Stored Integer
  Bus Creator : BusCreator  Inputs=7  OutDataTypeStr=Bus: CAN_MESSAGE_BUS  NonVirtualBus=on
  Bus Creator2 : BusCreator  Inputs=10
  Bus Selector : BusSelector  OutputSignals=AUTO_LiveCnt2
  Bus Selector1 : BusSelector  OutputSignals=AUTO_CheckSum2,AUTO_LiveCnt2,AUTO_PtoSpd,AUTO_Shutdown,AUTO_SuspMode,AUTO_Valve1,AUTO_Valve2,AUTO_Valve3,AUTO_Valve4
  Compare To Constant : simulink/Logic and Bit Operations/Compare To Constant  relop=>=  const=1  OutDataTypeStr=boolean
  Constant : Constant  OutDataTypeStr=uint8
  Constant1 : Constant  OutDataTypeStr=uint8
  Constant2 : Constant  Value=0
  Constant4 : Constant  Value=0  OutDataTypeStr=uint8
  Constant5 : Constant  Value=0  OutDataTypeStr=uint8
  Data Store Read : DataStoreRead  DataStoreName=Cnt_AUTO2
  Data Store Write : DataStoreWrite  DataStoreName=Cnt_AUTO2
  Data Type Conversion{,14..15,17} (4 alike) : DataTypeConversion  OutDataTypeStr=uint8
  Data Type Conversion18 : DataTypeConversion  OutDataTypeStr=uint32
  Data Type Conversion19 : DataTypeConversion  OutDataTypeStr=double
  Data Type Conversion8 : DataTypeConversion
  Demux : Demux  Outputs=8
  If : If
  If Action Subsystem : Subsystem  TreatAsAtomicUnit=on
  Manual Switch : ManualSwitch
  Merge : Merge
  Subsystem : Subsystem
  Unit Delay : UnitDelay  SampleTime=-1
  Message : Outport
  wires:
  Constant4/1 -> Data Type Conversion15/1
  length/1 -> Data Type Conversion14/1
  Data Type Conversion18/1 -> Bus Creator/5  "ID"
  Constant1/1 -> Data Type Conversion/1
  Constant5/1 -> Data Type Conversion17/1
  ID/1 -> Data Type Conversion18/1
  Data Type Conversion19/1 -> Bus Creator/6  "Timestamp"
  timestamp/1 -> Data Type Conversion19/1
  Data Type Conversion17/1 -> Bus Creator/4  "Error"
  Data Type Conversion/1 -> Bus Creator/1  "Extended"
  Data Type Conversion14/1 -> Bus Creator/2  "Length"
  Data Type Conversion15/1 -> Bus Creator/3  "Remote"
  Add/1 -> Data Store Write/1
  Constant/1 -> Add/2
  Data Store Read/1 -> Add/1
  If/1 -> If Action Subsystem/Action
  Unit Delay/1 -> If Action Subsystem/1(In1)
  Subsystem/1(Out1) -> Merge/2
  Bus Selector/1 -> [LiveCounter]  "<AUTO_LiveCnt2>"
  If Action Subsystem/1(Out1) -> Merge/1
  If/2 -> Subsystem/Action
  [checkSumFlg] -> Data Type Conversion8/1
  Data Type Conversion8/1 -> If/1
  Merge/1 -> Bus Selector1/1, Unit Delay/1, Bus Selector/1
  Bus Creator2/1 -> Message/1
  [PacketLossFlg] -> Bus Creator2/10  "PacketLossFlg"
  Bus Selector1/1 -> Bus Creator2/1  "<AUTO_CheckSum2>"
  Bus Selector1/2 -> Bus Creator2/2  "<AUTO_LiveCnt2>"
  Bus Selector1/3 -> Bus Creator2/3  "<AUTO_PtoSpd>"
  Bus Selector1/4 -> Bus Creator2/4  "<AUTO_Shutdown>"
  Bus Selector1/5 -> Bus Creator2/5  "<AUTO_SuspMode>"
  Bus Selector1/6 -> Bus Creator2/6  "<AUTO_Valve1>"
  Bus Selector1/7 -> Bus Creator2/7  "<AUTO_Valve2>"
  Bus Selector1/8 -> Bus Creator2/8  "<AUTO_Valve3>"
  Bus Selector1/9 -> Bus Creator2/9  "<AUTO_Valve4>"
  Demux/2 -> Bitwise XOR/2
  Bitwise XOR/1 -> Add1/1
  Auto PacketLoss/1(PacketLossFlg) -> [PacketLossFlg]  "PacketLossFlg"
  [checkSumFlg] -> Auto PacketLoss/2(CheckSumFlg)
  [LiveCounter] -> Auto PacketLoss/1(LiveCnt)
  Add1/1 -> Compare To Constant/1
  Demux/4 -> Bitwise XOR/4
  Demux/8 -> Add1/2
  Demux/3 -> Bitwise XOR/3
  Demux/7 -> Bitwise XOR/7
  Demux/6 -> Bitwise XOR/6
  Manual Switch/1 -> [checkSumFlg]
  Demux/1 -> Bitwise XOR/1
  data/1 -> Demux/1, Bus Creator/7  "Data"
  Demux/5 -> Bitwise XOR/5
  [checkSumFlg] -> Subsystem/1(In1)
  Bus Creator/1 -> Subsystem/2(CAN_Msg_In)  "CAN_Msg_In"
  Constant2/1 -> Manual Switch/1
  Compare To Constant/1 -> Manual Switch/2

== system VehCtrl20260630_18B/SigIn/CAN0/AUTO3/UNPACK ==
  ID : Inport
  data : Inport  Port=2
  length : Inport  Port=3
  timestamp : Inport  Port=4
  Action Port : ActionPort  ActionType=case
  Add : Sum
  Add1 : Sum  Inputs=+-
  Auto PacketLoss : Stateflow chart  TreatAsAtomicUnit=on
  Bitwise XOR : simulink/Logic and Bit Operations/Bitwise Operator  logicop=XOR  UseBitMask=off  NumInputPorts=7  BitMask=bin2dec('11011001')  BitMaskRealWorld=Stored Integer
  Bus Creator : BusCreator  Inputs=7  OutDataTypeStr=Bus: CAN_MESSAGE_BUS  NonVirtualBus=on
  Bus Creator2 : BusCreator  Inputs=7
  Bus Selector : BusSelector  OutputSignals=AUTO_LiveCnt1
  Bus Selector1 : BusSelector  OutputSignals=AUTO_CheckSum1,AUTO_LiveCnt1,AUTO_TrqCmdFL,AUTO_TrqCmdFR,AUTO_TrqCmdRL,AUTO_TrqCmdRR
  Compare To Constant : simulink/Logic and Bit Operations/Compare To Constant  relop=>=  const=1  OutDataTypeStr=boolean
  Constant : Constant  OutDataTypeStr=uint8
  Constant1 : Constant  OutDataTypeStr=uint8
  Constant2 : Constant  Value=0
  Constant4 : Constant  Value=0  OutDataTypeStr=uint8
  Constant5 : Constant  Value=0  OutDataTypeStr=uint8
  Data Store Read : DataStoreRead  DataStoreName=Cnt_AUTO3
  Data Store Write : DataStoreWrite  DataStoreName=Cnt_AUTO3
  Data Type Conversion{,14..15,17} (4 alike) : DataTypeConversion  OutDataTypeStr=uint8
  Data Type Conversion1 : DataTypeConversion
  Data Type Conversion18 : DataTypeConversion  OutDataTypeStr=uint32
  Data Type Conversion19 : DataTypeConversion  OutDataTypeStr=double
  Demux : Demux  Outputs=8
  If : If
  If Action Subsystem : Subsystem  TreatAsAtomicUnit=on
  Manual Switch : ManualSwitch
  Merge : Merge
  Subsystem : Subsystem
  Unit Delay : UnitDelay  SampleTime=-1
  Message : Outport
  wires:
  Compare To Constant/1 -> Manual Switch/2
  Constant2/1 -> Manual Switch/1
  Bus Creator/1 -> Subsystem/2(CAN_Msg_In)  "CAN_Msg_In"
  [checkSumFlg] -> Subsystem/1(In1)
  [PacketLossFlg] -> Bus Creator2/7  "PacketLossFlg"
  Bus Creator2/1 -> Message/1
  [LiveCounter] -> Auto PacketLoss/1(LiveCnt)
  [checkSumFlg] -> Auto PacketLoss/2(CheckSumFlg)
  Auto PacketLoss/1(PacketLossFlg) -> [PacketLossFlg]  "PacketLossFlg"
  Bus Selector1/5 -> Bus Creator2/5  "<AUTO_TrqCmdRL>"
  Bus Selector1/4 -> Bus Creator2/4  "<AUTO_TrqCmdFR>"
  Bus Selector1/3 -> Bus Creator2/3  "<AUTO_TrqCmdFL>"
  Bus Selector1/2 -> Bus Creator2/2  "<AUTO_LiveCnt1>"
  Bus Selector1/1 -> Bus Creator2/1  "<AUTO_CheckSum1>"
  Merge/1 -> Bus Selector/1, Unit Delay/1, Bus Selector1/1
  Data Type Conversion1/1 -> If/1
  [checkSumFlg] -> Data Type Conversion1/1
  If/2 -> Subsystem/Action
  If Action Subsystem/1(Out1) -> Merge/1
  Bus Selector/1 -> [LiveCounter]  "<AUTO_LiveCnt1>"
  Subsystem/1(Out1) -> Merge/2
  Unit Delay/1 -> If Action Subsystem/1(In1)
  If/1 -> If Action Subsystem/Action
  Demux/1 -> Bitwise XOR/1
  Demux/5 -> Bitwise XOR/5
  data/1 -> Bus Creator/7, Demux/1  "Data"
  Manual Switch/1 -> [checkSumFlg]
  Demux/6 -> Bitwise XOR/6
  Demux/7 -> Bitwise XOR/7
  Demux/3 -> Bitwise XOR/3
  Add1/1 -> Compare To Constant/1
  Demux/8 -> Add1/2
  Demux/4 -> Bitwise XOR/4
  Bitwise XOR/1 -> Add1/1
  Demux/2 -> Bitwise XOR/2
  Add/1 -> Data Store Write/1
  Constant/1 -> Add/2
  Data Store Read/1 -> Add/1
  Data Type Conversion15/1 -> Bus Creator/3  "Remote"
  Data Type Conversion14/1 -> Bus Creator/2  "Length"
  Data Type Conversion/1 -> Bus Creator/1  "Extended"
  Data Type Conversion17/1 -> Bus Creator/4  "Error"
  timestamp/1 -> Data Type Conversion19/1
  Data Type Conversion19/1 -> Bus Creator/6  "Timestamp"
  ID/1 -> Data Type Conversion18/1
  Constant5/1 -> Data Type Conversion17/1
  Constant1/1 -> Data Type Conversion/1
  Data Type Conversion18/1 -> Bus Creator/5  "ID"
  length/1 -> Data Type Conversion14/1
  Constant4/1 -> Data Type Conversion15/1
  Bus Selector1/6 -> Bus Creator2/6  "<AUTO_TrqCmdRR>"
